simulink library "lib_FDM"  (R2019b)
settings: Solver=VariableStepAuto  StartTime=0.0  StopTime=10.0  RelTol=1e-3
values from neighbouring files (symbols this model uses):
  d = config.d_m    [computeTF.m]
undefined symbols (not defined in the file or in its folder): c_b_WGS, c_flat, c_grav, c_rot, c_rsma, Cd0, Cdcl, Cdcl2, Cl0, Cla, Cld, Cma, Cmd, Cmq, Cnb, Cnd, Cnr, Cra, Crd, Crp, Cy0, Cyb, Cyd, dmdt, Earth, HIL_Data, InitThrust, launchPos, me, mf, mp, Sref, tb, TF, theta0, WGS84
libraries: simulink_extras x14, $bdroot x7, simulink x5, lib_Fin_Deflections x3, aerolibasang x2, sharedtransform x1, aerolibtransform2 x1, aerolibbdyn x1, aerolibatmos2 x1, aerolibutil x1, aerolib6dof2 x1
(part 3 of 8)

== system lib_FDM/FDM/FDM_Basic/State_Integration/VEL_Integrator ==
  Simulation_Control : Inport  OutDataTypeStr=Bus: Simulation_Ctrl_Bus
  Initial_States : Inport  Port=2  OutDataTypeStr=Bus: States_Bus
  ax_mDs2 : Inport  Port=3
  ay_mDs2 : Inport  Port=4
  az_mDs2 : Inport  Port=5
  Bus Selector : BusSelector  OutputSignals=run,reset
  Bus Selector1 : BusSelector  OutputSignals=Rigid_Body_States.Translation_States.VEL_u_K_R_E_B_mDs
  Bus Selector2 : BusSelector  OutputSignals=Rigid_Body_States.Translation_States.VEL_v_K_R_E_B_mDs
  Bus Selector3 : BusSelector  OutputSignals=Rigid_Body_States.Translation_States.VEL_w_K_R_E_B_mDs
  Data Type Conversion : DataTypeConversion  OutDataTypeStr=double
  Integrator : Integrator  ExternalReset=rising  InitialConditionSource=external
  Integrator1 : Integrator  ExternalReset=rising  InitialConditionSource=external
  Integrator2 : Integrator  ExternalReset=rising  InitialConditionSource=external
  Product : Product
  Product1 : Product
  Product2 : Product
  u_mDs : Outport  VectorParamsAs1DForOutWhenUnconnected=off
  v_mDs : Outport  Port=2  VectorParamsAs1DForOutWhenUnconnected=off
  w_mDs : Outport  Port=3  VectorParamsAs1DForOutWhenUnconnected=off
  wires:
  Simulation_Control/1 -> Bus Selector/1
  Bus Selector/1 -> Data Type Conversion/1  "<run>"
  Data Type Conversion/1 -> Product/2, Product1/2, Product2/2
  Product/1 -> Integrator/1
  az_mDs2/1 -> Product2/1
  ay_mDs2/1 -> Product1/1
  ax_mDs2/1 -> Product/1
  Bus Selector/2 -> Integrator2/2, Integrator1/2, Integrator/2  "<reset>"
  Bus Selector1/1 -> Integrator/3  "<VEL_u_K_R_E_B_mDs>"
  Product1/1 -> Integrator1/1
  Initial_States/1 -> Bus Selector3/1, Bus Selector2/1, Bus Selector1/1
  Product2/1 -> Integrator2/1
  Integrator/1 -> u_mDs/1  "u"
  Integrator1/1 -> v_mDs/1  "v"
  Integrator2/1 -> w_mDs/1  "w"
  Bus Selector3/1 -> Integrator2/3  "<VEL_w_K_R_E_B_mDs>"
  Bus Selector2/1 -> Integrator1/3  "<VEL_v_K_R_E_B_mDs>"

== system lib_FDM/FDM/FDM_Linear/Motion_Kinematics/Drag ==
  alpha : Inport
  beta : Inport  Port=2
  Enable : EnablePort
  Constant : Constant  Value=-1
  Constant1 : Constant  Value=-1
  Constant2 : Constant  Value=-1
  Terminator : Terminator
  Terminator1 : Terminator
  acc_x_drag_mDs2 : Outport  OutputWhenDisabled=reset  InitialOutput=0  VectorParamsAs1DForOutWhenUnconnected=off
  acc_y_drag_mDs2 : Outport  Port=2  OutputWhenDisabled=reset  InitialOutput=0  VectorParamsAs1DForOutWhenUnconnected=off
  acc_z_drag_mDs2 : Outport  Port=3  OutputWhenDisabled=reset  InitialOutput=0  VectorParamsAs1DForOutWhenUnconnected=off
  wires:
  alpha/1 -> Terminator/1
  beta/1 -> Terminator1/1
  Constant/1 -> acc_x_drag_mDs2/1
  Constant1/1 -> acc_y_drag_mDs2/1
  Constant2/1 -> acc_z_drag_mDs2/1

== system lib_FDM/FDM/FDM_Linear/Motion_Kinematics/Gravity ==
  note: derived from transformation matrix NED to Body
  note: for decoupling, set phi to zero??!!!
  phi : Inport
  theta : Inport  Port=2
  psi : Inport  Port=3
  Enable : EnablePort
  Constant1 : Constant  Value=FDM.Environment_Data.gravity_mDs2
  MATLAB Function : MATLAB Function  TreatAsAtomicUnit=on
  acc_x_grav_mDs : Outport  OutputWhenDisabled=reset  InitialOutput=0  VectorParamsAs1DForOutWhenUnconnected=off
  acc_y_grav_mDs : Outport  Port=2  OutputWhenDisabled=reset  InitialOutput=0  VectorParamsAs1DForOutWhenUnconnected=off
  acc_z_grav_mDs : Outport  Port=3  OutputWhenDisabled=reset  InitialOutput=0  VectorParamsAs1DForOutWhenUnconnected=off
  wires:
  Constant1/1 -> MATLAB Function/1(g)
  phi/1 -> MATLAB Function/2(phi)
  theta/1 -> MATLAB Function/3(theta)
  psi/1 -> MATLAB Function/4(psi)
  MATLAB Function/1(acc_x) -> acc_x_grav_mDs/1
  MATLAB Function/2(acc_y) -> acc_y_grav_mDs/1
  MATLAB Function/3(acc_z) -> acc_z_grav_mDs/1

== system lib_FDM/FDM/FDM_Linear/Motion_Kinematics/NED2PosWGS84Dot ==
  note: derived from Scriptum
  mue_rad : Inport
  h_m : Inport  Port=2
  x_dot_NED_mDs : Inport  Port=3
  y_dot_NED_mDs : Inport  Port=4
  z_dot_NED_mDs : Inport  Port=5
  MATLAB Function : MATLAB Function  TreatAsAtomicUnit=on
  lambda_dot_radDs : Outport  VectorParamsAs1DForOutWhenUnconnected=off
  mue_dot_radDs : Outport  Port=2  VectorParamsAs1DForOutWhenUnconnected=off
  h_dot_mDs : Outport  Port=3  VectorParamsAs1DForOutWhenUnconnected=off
  wires:
  h_m/1 -> MATLAB Function/5(h)
  mue_rad/1 -> MATLAB Function/4(mue)
  z_dot_NED_mDs/1 -> MATLAB Function/3(z_dot_NED)
  y_dot_NED_mDs/1 -> MATLAB Function/2(y_dot_NED)
  x_dot_NED_mDs/1 -> MATLAB Function/1(x_dot_NED)
  MATLAB Function/3(h_dot) -> h_dot_mDs/1
  MATLAB Function/2(mue_dot) -> mue_dot_radDs/1
  MATLAB Function/1(lambda_dot) -> lambda_dot_radDs/1

== system lib_FDM/FDM/FDM_Linear/Motion_Kinematics/Propulsion ==
  Motor_Ignition_flg : Inport
  Enable : EnablePort
  Add : Sum  Inputs=-+
  Clock : Clock
  Compare To Constant : simulink/Logic and Bit Operations/Compare To Constant  relop=<  const=FDM.Configuration_Data.Propulsion.burntime_s  OutDataTypeStr=boolean
  Logical Operator : Logic  Operator=NOT  AllPortsSameDT=off  OutDataTypeStr=boolean
  Logical Operator1 : Logic  Operator=OR  AllPortsSameDT=off  OutDataTypeStr=boolean
  Logical Operator2 : Logic  AllPortsSameDT=off  OutDataTypeStr=boolean
  Subsystem : Subsystem
  hold_time : Subsystem
  lock : Memory
  F_x_prop_N : Outport  VectorParamsAs1DForOutWhenUnconnected=off
  motor_state_perc_dot : Outport  Port=2  OutputWhenDisabled=reset  InitialOutput=0  VectorParamsAs1DForOutWhenUnconnected=off
  wires:
  Motor_Ignition_flg/1 -> Logical Operator1/1
  Logical Operator1/1 -> lock/1, Logical Operator/1, Logical Operator2/1
  lock/1 -> Logical Operator1/2
  Logical Operator/1 -> hold_time/Enable
  hold_time/1(exec_time_hold_s) -> Add/1
  Clock/1 -> Add/2
  Add/1 -> Compare To Constant/1, Subsystem/1(runtime)
  Subsystem/1(thrust) -> F_x_prop_N/1
  Subsystem/2(state_percentage_change) -> motor_state_perc_dot/1
  Compare To Constant/1 -> Logical Operator2/2
  Logical Operator2/1 -> Subsystem/Enable

== system lib_FDM/FDM/FDM_Linear/Motion_Kinematics/pqr2EulerDot ==
  ATT : Inport  OutDataTypeStr=Bus: ATT_Euler_Bus
  p : Inport  Port=2
  q : Inport  Port=3
  r : Inport  Port=4
  Add : Sum  Inputs=+++
  Add1 : Sum
  Add2 : Sum
  Bus Selector : BusSelector  OutputSignals=ATT_Phi_rad,ATT_Theta_rad
  Divide : Product  Inputs=*/
  Divide1 : Product  Inputs=*/
  Fcn1 : Fcn  Expr=-sin(u)
  Fcn{6,8,10..12} (5 alike) : Fcn  Expr=cos(u)
  Fcn4 : Fcn  Expr=sin(u)
  Fcn5 : Fcn  Expr=tan(u)
  Fcn7 : Fcn  Expr=tan(u)
  Fcn9 : Fcn  Expr=sin(u)
  Multiply{,1..7} (8 alike) : Product
  phi_dot : Outport  VectorParamsAs1DForOutWhenUnconnected=off
  theta_dot : Outport  Port=2  VectorParamsAs1DForOutWhenUnconnected=off
  psi_dot : Outport  Port=3  VectorParamsAs1DForOutWhenUnconnected=off
  wires:
  ATT/1 -> Bus Selector/1
  Add2/1 -> psi_dot/1
  Add1/1 -> theta_dot/1
  Add/1 -> phi_dot/1
  Fcn4/1 -> Multiply/1
  Fcn5/1 -> Multiply/2
  p/1 -> Add/1
  Bus Selector/1 -> Fcn1/1, Fcn8/1, Fcn6/1, Fcn4/1, Fcn11/1, Fcn9/1  "<ATT_Phi_rad>"
  Bus Selector/2 -> Fcn7/1, Fcn5/1, Fcn12/1, Fcn10/1  "<ATT_Theta_rad>"
  Fcn6/1 -> Multiply1/1
  Fcn7/1 -> Multiply1/2
  Fcn9/1 -> Divide/1
  Fcn10/1 -> Divide/2
  Fcn11/1 -> Divide1/1
  Fcn12/1 -> Divide1/2
  Multiply/1 -> Multiply2/2
  q/1 -> Multiply2/1, Multiply6/1, Multiply4/2
  Multiply2/1 -> Add/2
  Multiply1/1 -> Multiply3/2
  r/1 -> Multiply3/1, Multiply7/1, Multiply5/2
  Multiply3/1 -> Add/3
  Fcn8/1 -> Multiply4/1
  Fcn1/1 -> Multiply5/1
  Multiply4/1 -> Add1/1
  Multiply5/1 -> Add1/2
  Divide/1 -> Multiply6/2
  Divide1/1 -> Multiply7/2
  Multiply6/1 -> Add2/1
  Multiply7/1 -> Add2/2

== system lib_FDM/FDM/FDM_Linear/Motion_Kinematics/uvw2PosNEDDot ==
  note: for decoupling, set phi to zero??!!!
  note: derived from Rotation Matrix Body Frame to NED Frame
  u : Inport
  v : Inport  Port=2
  w : Inport  Port=3
  ATT : Inport  Port=4  OutDataTypeStr=Bus: ATT_Euler_Bus
  Bus Selector : BusSelector  OutputSignals=ATT_Phi_rad,ATT_Theta_rad,ATT_Psi_rad
  MATLAB Function : MATLAB Function  TreatAsAtomicUnit=on
  MATLAB Function1 : MATLAB Function  TreatAsAtomicUnit=on
  MATLAB Function2 : MATLAB Function  TreatAsAtomicUnit=on
  x_dot_mDs : Outport  VectorParamsAs1DForOutWhenUnconnected=off
  y_dot_mDs : Outport  Port=2  VectorParamsAs1DForOutWhenUnconnected=off
  z_dot_mDs : Outport  Port=3  VectorParamsAs1DForOutWhenUnconnected=off
  wires:
  ATT/1 -> Bus Selector/1
  u/1 -> MATLAB Function2/1(u), MATLAB Function1/1(u), MATLAB Function/1(u)
  v/1 -> MATLAB Function2/2(v), MATLAB Function1/2(v), MATLAB Function/2(v)
  w/1 -> MATLAB Function2/3(w), MATLAB Function1/3(w), MATLAB Function/3(w)
  Bus Selector/1 -> MATLAB Function2/4(phi), MATLAB Function1/4(phi), MATLAB Function/4(phi)  "<ATT_Phi_rad>"
  Bus Selector/2 -> MATLAB Function2/5(theta), MATLAB Function1/5(theta), MATLAB Function/5(theta)  "<ATT_Theta_rad>"
  Bus Selector/3 -> MATLAB Function1/6(psi), MATLAB Function/6(psi)  "<ATT_Psi_rad>"
  MATLAB Function/1(N_dot) -> x_dot_mDs/1
  MATLAB Function1/1(E_dot) -> y_dot_mDs/1
  MATLAB Function2/1(D_dot) -> z_dot_mDs/1

== system lib_FDM/FDM/FDM_Linear/State_Integration/ATT_Integration ==
  Simulation_Control : Inport  OutDataTypeStr=Bus: Simulation_Ctrl_Bus
  Initial_States : Inport  Port=2  OutDataTypeStr=Bus: States_Bus
  phi_dot_radDs : Inport  Port=3
  theta_dot_radDs : Inport  Port=4
  psi_dot_radDs : Inport  Port=5
  Bus Selector : BusSelector  OutputSignals=run,reset
  Bus Selector1 : BusSelector  OutputSignals=Rigid_Body_States.Attitude_States.ATT_Euler.ATT_Phi_rad
  Bus Selector2 : BusSelector  OutputSignals=Rigid_Body_States.Attitude_States.ATT_Euler.ATT_Theta_rad
  Bus Selector3 : BusSelector  OutputSignals=Rigid_Body_States.Attitude_States.ATT_Euler.ATT_Psi_rad
  Data Type Conversion : DataTypeConversion  OutDataTypeStr=double
  Integrator : Integrator  ExternalReset=rising  InitialConditionSource=external
  Integrator1 : Integrator  ExternalReset=rising  InitialConditionSource=external
  Integrator2 : Integrator  ExternalReset=rising  InitialConditionSource=external
  Product : Product
  Product1 : Product
  Product2 : Product
  phi_rad : Outport  VectorParamsAs1DForOutWhenUnconnected=off
  theta_rad : Outport  Port=2  VectorParamsAs1DForOutWhenUnconnected=off
  psi_rad : Outport  Port=3  VectorParamsAs1DForOutWhenUnconnected=off
  wires:
  Simulation_Control/1 -> Bus Selector/1
  Bus Selector/1 -> Data Type Conversion/1  "<run>"
  Data Type Conversion/1 -> Product/2, Product1/2, Product2/2
  Product/1 -> Integrator/1
  psi_dot_radDs/1 -> Product2/1
  theta_dot_radDs/1 -> Product1/1
  phi_dot_radDs/1 -> Product/1
  Bus Selector/2 -> Integrator2/2, Integrator1/2, Integrator/2  "<reset>"
  Bus Selector1/1 -> Integrator/3  "<ATT_Phi_rad>"
  Product1/1 -> Integrator1/1
  Initial_States/1 -> Bus Selector3/1, Bus Selector2/1, Bus Selector1/1
  Product2/1 -> Integrator2/1
  Integrator/1 -> phi_rad/1
  Integrator1/1 -> theta_rad/1
  Integrator2/1 -> psi_rad/1
  Bus Selector3/1 -> Integrator2/3  "<ATT_Psi_rad>"
  Bus Selector2/1 -> Integrator1/3  "<ATT_Theta_rad>"

== system lib_FDM/FDM/FDM_Linear/State_Integration/Mass_Balance ==
  note: linear interpolation between initial and burnout values of inertia and mass
  motor_state_perc : Inport
  Add{,1..3} (4 alike) : Sum
  Constant : Constant  Value=FDM.Configuration_Data.mass_preburn_kg-FDM.Configuration_Data.mass_kg
  Constant1 : Constant  Value=FDM.Configuration_Data.mass_kg
  Constant2 : Constant  Value=FDM.Configuration_Data.I_x_kgDm2
  Constant3 : Constant  Value=FDM.Configuration_Data.I_x_preburn_kgDm2-FDM.Configuration_Data.I_x_kgDm2
  Constant4 : Constant  Value=FDM.Configuration_Data.I_y_kgDm2
  Constant5 : Constant  Value=FDM.Configuration_Data.I_y_preburn_kgDm2-FDM.Configuration_Data.I_y_kgDm2
  Constant6 : Constant  Value=FDM.Configuration_Data.I_z_kgDm2
  Constant7 : Constant  Value=FDM.Configuration_Data.I_z_preburn_kgDm2-FDM.Configuration_Data.I_z_kgDm2
  Multiply{,1..3} (4 alike) : Product
  mass_kg : Outport  VectorParamsAs1DForOutWhenUnconnected=off
  I_x_kgm2 : Outport  Port=2  VectorParamsAs1DForOutWhenUnconnected=off
  I_y_kgm2 : Outport  Port=3  VectorParamsAs1DForOutWhenUnconnected=off
  I_z_kgm2 : Outport  Port=4  VectorParamsAs1DForOutWhenUnconnected=off
  wires:
  Constant1/1 -> Add/1
  Constant/1 -> Multiply/2
  Multiply/1 -> Add/2
  motor_state_perc/1 -> Multiply1/1, Multiply2/1, Multiply3/1, Multiply/1
  Add/1 -> mass_kg/1
  Constant3/1 -> Multiply1/2
  Multiply1/1 -> Add1/2
  Constant2/1 -> Add1/1
  Constant5/1 -> Multiply2/2
  Constant4/1 -> Add2/1
  Multiply2/1 -> Add2/2
  Constant6/1 -> Add3/1
  Constant7/1 -> Multiply3/2
  Multiply3/1 -> Add3/2
  Add1/1 -> I_x_kgm2/1
  Add2/1 -> I_y_kgm2/1
  Add3/1 -> I_z_kgm2/1

== system lib_FDM/FDM/FDM_Linear/State_Integration/Motor_State_Integration ==
  Simulation_Control : Inport  OutDataTypeStr=Bus: Simulation_Ctrl_Bus
  Initial_States : Inport  Port=2  OutDataTypeStr=Bus: States_Bus
  motor_state_dot_percDs : Inport  Port=3
  Bus Selector2 : BusSelector  OutputSignals=Airframe_States.motor_state_perc
  Bus Selector3 : BusSelector  OutputSignals=run,reset
  Data Type Conversion : DataTypeConversion  OutDataTypeStr=double
  Integrator : Integrator  ExternalReset=rising  InitialConditionSource=external
  Multiply : Product
  motor_state_perc : Outport  VectorParamsAs1DForOutWhenUnconnected=off
  wires:
  Bus Selector2/1 -> Integrator/3  "<motor_state_perc>"
  Bus Selector3/2 -> Integrator/2  "<reset>"
  Bus Selector3/1 -> Data Type Conversion/1  "<run>"
  motor_state_dot_percDs/1 -> Multiply/1
  Integrator/1 -> motor_state_perc/1
  Multiply/1 -> Integrator/1
  Simulation_Control/1 -> Bus Selector3/1
  Initial_States/1 -> Bus Selector2/1
  Data Type Conversion/1 -> Multiply/2

== system lib_FDM/FDM/FDM_Linear/State_Integration/POS_NED_Integrator ==
  Simulation_Control : Inport  OutDataTypeStr=Bus: Simulation_Ctrl_Bus
  Initial_States : Inport  Port=2  OutDataTypeStr=Bus: States_Bus
  x_dot_mDs : Inport  Port=3
  y_dot_mDs : Inport  Port=4
  z_dot_mDs : Inport  Port=5
  Bus Selector : BusSelector  OutputSignals=run,reset
  Bus Selector1 : BusSelector  OutputSignals=Rigid_Body_States.Position_States.POS_NED.POS_x_NED_m
  Bus Selector2 : BusSelector  OutputSignals=Rigid_Body_States.Position_States.POS_NED.POS_y_NED_m
  Bus Selector3 : BusSelector  OutputSignals=Rigid_Body_States.Position_States.POS_NED.POS_z_NED_m
  Data Type Conversion : DataTypeConversion  OutDataTypeStr=double
  Integrator : Integrator  ExternalReset=rising  InitialConditionSource=external
  Integrator1 : Integrator  ExternalReset=rising  InitialConditionSource=external
  Integrator2 : Integrator  ExternalReset=rising  InitialConditionSource=external
  Product : Product
  Product1 : Product
  Product2 : Product
  x_m : Outport  VectorParamsAs1DForOutWhenUnconnected=off
  y_m : Outport  Port=2  VectorParamsAs1DForOutWhenUnconnected=off
  z_m : Outport  Port=3  VectorParamsAs1DForOutWhenUnconnected=off
  wires:
  Simulation_Control/1 -> Bus Selector/1
  Bus Selector/1 -> Data Type Conversion/1  "<run>"
  Data Type Conversion/1 -> Product/2, Product1/2, Product2/2
  Product/1 -> Integrator/1
  z_dot_mDs/1 -> Product2/1
  y_dot_mDs/1 -> Product1/1
  x_dot_mDs/1 -> Product/1
  Bus Selector/2 -> Integrator2/2, Integrator1/2, Integrator/2  "<reset>"
  Bus Selector1/1 -> Integrator/3  "<POS_x_NED_m>"
  Product1/1 -> Integrator1/1
  Initial_States/1 -> Bus Selector3/1, Bus Selector2/1, Bus Selector1/1
  Product2/1 -> Integrator2/1
  Integrator/1 -> x_m/1
  Integrator1/1 -> y_m/1
  Integrator2/1 -> z_m/1
  Bus Selector3/1 -> Integrator2/3  "<POS_z_NED_m>"
  Bus Selector2/1 -> Integrator1/3  "<POS_y_NED_m>"

== system lib_FDM/FDM/FDM_Linear/State_Integration/POS_WGS84_Integrator ==
  Simulation_Control : Inport  OutDataTypeStr=Bus: Simulation_Ctrl_Bus
  Initial_States : Inport  Port=2  OutDataTypeStr=Bus: States_Bus
  lambda_dot_radDs : Inport  Port=3
  mue_dot_radDs : Inport  Port=4
  h_dot_mDs : Inport  Port=5
  Bus Selector : BusSelector  OutputSignals=run,reset
  Bus Selector1 : BusSelector  OutputSignals=Rigid_Body_States.Position_States.POS_WGS84.POS_lambda_WGS84_rad
  Bus Selector2 : BusSelector  OutputSignals=Rigid_Body_States.Position_States.POS_WGS84.POS_mue_WGS84_rad
  Bus Selector3 : BusSelector  OutputSignals=Rigid_Body_States.Position_States.POS_WGS84.POS_h_WGS84_m
  Data Type Conversion : DataTypeConversion  OutDataTypeStr=double
  Integrator : Integrator  ExternalReset=rising  InitialConditionSource=external
  Integrator1 : Integrator  ExternalReset=rising  InitialConditionSource=external
  Integrator2 : Integrator  ExternalReset=rising  InitialConditionSource=external
  Product : Product
  Product1 : Product
  Product2 : Product
  lambda_rad : Outport  VectorParamsAs1DForOutWhenUnconnected=off
  mue_rad : Outport  Port=2  VectorParamsAs1DForOutWhenUnconnected=off
  h_m : Outport  Port=3  VectorParamsAs1DForOutWhenUnconnected=off
  wires:
  Simulation_Control/1 -> Bus Selector/1
  Bus Selector/1 -> Data Type Conversion/1  "<run>"
  Data Type Conversion/1 -> Product/2, Product1/2, Product2/2
  Product/1 -> Integrator/1
  h_dot_mDs/1 -> Product2/1
  mue_dot_radDs/1 -> Product1/1
  lambda_dot_radDs/1 -> Product/1
  Bus Selector/2 -> Integrator2/2, Integrator1/2, Integrator/2  "<reset>"
  Bus Selector1/1 -> Integrator/3  "<POS_lambda_WGS84_rad>"
  Product1/1 -> Integrator1/1
  Initial_States/1 -> Bus Selector3/1, Bus Selector2/1, Bus Selector1/1
  Product2/1 -> Integrator2/1
  Integrator/1 -> lambda_rad/1
  Integrator1/1 -> mue_rad/1
  Integrator2/1 -> h_m/1
  Bus Selector3/1 -> Integrator2/3  "<POS_h_WGS84_m>"
  Bus Selector2/1 -> Integrator1/3  "<POS_mue_WGS84_rad>"

== system lib_FDM/FDM/FDM_Linear/State_Integration/VEL_Integrator ==
  Simulation_Control : Inport  OutDataTypeStr=Bus: Simulation_Ctrl_Bus
  Initial_States : Inport  Port=2  OutDataTypeStr=Bus: States_Bus
  ax_mDs2 : Inport  Port=3
  ay_mDs2 : Inport  Port=4
  az_mDs2 : Inport  Port=5
  Bus Selector : BusSelector  OutputSignals=run,reset
  Bus Selector1 : BusSelector  OutputSignals=Rigid_Body_States.Translation_States.VEL_u_K_R_E_B_mDs
  Bus Selector2 : BusSelector  OutputSignals=Rigid_Body_States.Translation_States.VEL_v_K_R_E_B_mDs
  Bus Selector3 : BusSelector  OutputSignals=Rigid_Body_States.Translation_States.VEL_w_K_R_E_B_mDs
  Data Type Conversion : DataTypeConversion  OutDataTypeStr=double
  Integrator : Integrator  ExternalReset=rising  InitialConditionSource=external
  Integrator1 : Integrator  ExternalReset=rising  InitialConditionSource=external
  Integrator2 : Integrator  ExternalReset=rising  InitialConditionSource=external
  Product : Product
  Product1 : Product
  Product2 : Product
  u_mDs : Outport  VectorParamsAs1DForOutWhenUnconnected=off
  v_mDs : Outport  Port=2  VectorParamsAs1DForOutWhenUnconnected=off
  w_mDs : Outport  Port=3  VectorParamsAs1DForOutWhenUnconnected=off
  wires:
  Simulation_Control/1 -> Bus Selector/1
  Bus Selector/1 -> Data Type Conversion/1  "<run>"
  Data Type Conversion/1 -> Product/2, Product1/2, Product2/2
  Product/1 -> Integrator/1
  az_mDs2/1 -> Product2/1
  ay_mDs2/1 -> Product1/1
  ax_mDs2/1 -> Product/1
  Bus Selector/2 -> Integrator2/2, Integrator1/2, Integrator/2  "<reset>"
  Bus Selector1/1 -> Integrator/3  "<VEL_u_K_R_E_B_mDs>"
  Product1/1 -> Integrator1/1
  Initial_States/1 -> Bus Selector3/1, Bus Selector2/1, Bus Selector1/1
  Product2/1 -> Integrator2/1
  Integrator/1 -> u_mDs/1  "u"
  Integrator1/1 -> v_mDs/1  "v"
  Integrator2/1 -> w_mDs/1  "w"
  Bus Selector3/1 -> Integrator2/3  "<VEL_w_K_R_E_B_mDs>"
  Bus Selector2/1 -> Integrator1/3  "<VEL_v_K_R_E_B_mDs>"

== system lib_FDM/FDM/FDM_Sophisticated/Subsystem/control_allocation ==
  fin_cmd : Inport
  Constant7 : Constant  Value=HIL_Data.FDM.soph.bus1.Tr4r3
  Product : Product  Multiplication=Matrix(*)
  siB_cmd : Outport  VectorParamsAs1DForOutWhenUnconnected=off
  wires:
  Constant7/1 -> Product/1
  fin_cmd/1 -> Product/2
  Product/1 -> siB_cmd/1  "siB_cmd"

== system lib_FDM/FDM/FDM_Sophisticated/aerodynamics/aerodynamic_via_lookup ==
  pBSB : Inport
  qdynB : Inport  Port=2
  MaB : Inport  Port=3
  alB : Inport  Port=4
  beB : Inport  Port=5
  hBE : Inport  Port=6
  wBIB_star : Inport  Port=7
  afinB : Inport  Port=8
  flag_I_prp : Inport  Port=9
  Bus Creator : BusCreator  Inputs=2
  calc_aero_coefficients : Subsystem
  calc_aero_for_mom : Subsystem
  calc_derivatives : Subsystem
  transform_rad2deg_al_be : Subsystem
  transform_rad2deg_fin : Subsystem
  transform_rad2deg_rates : Subsystem
  aero_bus : Outport  VectorParamsAs1DForOutWhenUnconnected=off
  wires:
  transform_rad2deg_al_be/2(beB_deg) -> calc_derivatives/4(beB)
  transform_rad2deg_al_be/1(alB_deg) -> calc_derivatives/3(alB)
  beB/1 -> transform_rad2deg_al_be/2(beB)
  afinB/1 -> transform_rad2deg_fin/1(afinB)
  qdynB/1 -> calc_aero_for_mom/3(qdynB)
  calc_aero_for_mom/2(MBAB) -> Bus Creator/2
  calc_aero_coefficients/6(Cn) -> calc_aero_for_mom/9(Cn)
  calc_aero_coefficients/1(Cx) -> calc_aero_for_mom/4(Cx)
  calc_aero_coefficients/5(Cm) -> calc_aero_for_mom/8(Cm)
  calc_derivatives/4(Cl_deriv) -> calc_aero_coefficients/4(Cl_deriv)
  calc_aero_coefficients/3(Cz) -> calc_aero_for_mom/6(Cz)
  hBE/1 -> calc_aero_for_mom/1(hBE), calc_derivatives/1(hBE)
  flag_I_prp/1 -> calc_aero_coefficients/13(flag_base_drag)
  calc_derivatives/6(Cn_deriv) -> calc_aero_coefficients/6(Cn_deriv)
  wBIB_star/1 -> transform_rad2deg_rates/1(wBIB_star)
  calc_derivatives/3(Cz_deriv) -> calc_aero_coefficients/3(Cz_deriv)
  pBSB/1 -> calc_aero_for_mom/2(pBSB)
  transform_rad2deg_rates/2(qBIB_star_deg) -> calc_aero_coefficients/11(qBIB_star)
  transform_rad2deg_rates/3(rBIB_star_deg) -> calc_aero_coefficients/12(rBIB_star)
  Bus Creator/1 -> aero_bus/1  "aero_bus"
  calc_aero_coefficients/2(Cy) -> calc_aero_for_mom/5(Cy)
  calc_derivatives/5(Cm_deriv) -> calc_aero_coefficients/5(Cm_deriv)
  calc_derivatives/2(Cy_deriv) -> calc_aero_coefficients/2(Cy_deriv)
  transform_rad2deg_rates/1(pBIB_star_deg) -> calc_aero_coefficients/10(pBIB_star)
  transform_rad2deg_fin/3(xiB_deg) -> calc_aero_coefficients/9(xiB_deg)
  transform_rad2deg_fin/2(zeB_deg) -> calc_aero_coefficients/8(zeB_deg), calc_derivatives/6(zeB_deg)
  alB/1 -> transform_rad2deg_al_be/1(alB)
  transform_rad2deg_fin/1(etB_deg) -> calc_derivatives/5(etB_deg), calc_aero_coefficients/7(etB_deg)
  calc_derivatives/1(Cx_deriv) -> calc_aero_coefficients/1(Cx_deriv)
  calc_aero_for_mom/1(FBAB) -> Bus Creator/1
  MaB/1 -> calc_derivatives/2(MaB)
  calc_aero_coefficients/4(Cl) -> calc_aero_for_mom/7(Cl)

== system lib_FDM/FDM/FDM_Sophisticated/aerodynamics/logic_base_drag ==
  env_glbl : Inport
  Bus Selector1 : BusSelector  OutputSignals=T_sim_glbl,T_sim_lnch
  Constant : Constant  Value=HIL_Data.FDM.soph.bus1.t_prp2(end)
  MATLAB Function : MATLAB Function  TreatAsAtomicUnit=on
  Subtract : Sum  Inputs=+-
  flag_base_drag : Outport  VectorParamsAs1DForOutWhenUnconnected=off
  wires:
  env_glbl/1 -> Bus Selector1/1
  Bus Selector1/2 -> Subtract/2  "<T_sim_lnch>"
  Bus Selector1/1 -> Subtract/1  "<T_sim_glbl>"
  MATLAB Function/1(flag_base_drag) -> flag_base_drag/1  "flag_base_drag"
  Constant/1 -> MATLAB Function/2(t_prp2)
  Subtract/1 -> MATLAB Function/1(u)

== system lib_FDM/FDM/FDM_Sophisticated/environment/WGS84_Gravitation ==
  lon : Inport  PortDimensions=1
  lat : Inport  Port=2  PortDimensions=1
  h : Inport  Port=3  PortDimensions=1
  Assertion : Assertion  AssertionFailFcn="error('WGS84 Gravitationsmodell: Die Werte des Eingangs \"h\" muessen groesser als 0 sein')"
  Assertion1 : Assertion  AssertionFailFcn="error('WGS84 Gravitationsmodell: Die Werte des Eingangs \"Long\" muessen zwischen -180 und +180 liegen')"
  Assertion2 : Assertion  AssertionFailFcn="error('WGS84 Gravitationsmodell: Die Werte des Eingangs \"Lat\" muessen zwischen -90 und +90 liegen')"
  Compare To Constant : simulink/Logic and Bit Operations/Compare To Constant  relop=>=  const=0  OutDataTypeStr=boolean
      settings: SourceProductName=ISim Simulink Block Set
  Interval Test : simulink/Logic and Bit Operations/Interval Test  IntervalClosedRight=on  uplimit=pi  IntervalClosedLeft=on  lowlimit=-pi  OutDataTypeStr=boolean
      settings: SourceProductName=ISim Simulink Block Set
  Interval Test1 : simulink/Logic and Bit Operations/Interval Test  IntervalClosedRight=on  uplimit=pi/2  IntervalClosedLeft=on  lowlimit=-pi/2  OutDataTypeStr=boolean
      settings: SourceProductName=ISim Simulink Block Set
  WGS84_2_ECEF : Subsystem
  WGS84_Gravity_Implementation : MATLAB Function  TreatAsAtomicUnit=on
  gE : Outport  PortDimensions=3  VectorParamsAs1DForOutWhenUnconnected=off
  wires:
  WGS84_Gravity_Implementation/1(gamma_R) -> gE/1  "gE"
  h/1 -> Compare To Constant/1, WGS84_2_ECEF/1(h)  "h"
  lon/1 -> WGS84_2_ECEF/2(lon), Interval Test/1, WGS84_Gravity_Implementation/3(long_rad)  "lon"
  lat/1 -> WGS84_2_ECEF/3(lat), Interval Test1/1, WGS84_Gravity_Implementation/2(lat_rad)  "lat"
  WGS84_2_ECEF/1(pE) -> WGS84_Gravity_Implementation/1(pE)  "pE"
  Compare To Constant/1 -> Assertion/1
  Interval Test/1 -> Assertion1/1
  Interval Test1/1 -> Assertion2/1

== system lib_FDM/FDM/FDM_Sophisticated/environment/atmosphere_static_ISO_2533 ==
  hBE : Inport
  env_glbl : Inport  Port=2
  Bus Creator1 : BusCreator  Inputs=6
  Bus Selector1 : BusSelector  OutputSignals=e_Tmp,e_pa
  Saturation : Saturate  UpperLimit=HIL_Data.FDM.soph.bus2.c_h_geope  LowerLimit=HIL_Data.FDM.soph.bus2.c_h_geop0
      settings: AttributesFormatString=|
      | %<UpperLimit>
      | %<LowerLimit>
  density : Subsystem
  geopot_height : Subsystem  mask{mean_earth_radius=HIL_Data.FDM.soph.bus2.c_r0}
      mask prompts: mean_earth_radius "Mean Earth Radius WGS 84 [m]"
      mask TypeOptions mean_earth_radius: mean_earth_radius/Value
  speed_of_sound : Subsystem
  tmp_and_pressure_ISO_2533 : Subsystem
  atm_stat : Outport  VectorParamsAs1DForOutWhenUnconnected=off
  wires:
  Saturation/1 -> tmp_and_pressure_ISO_2533/1(h_geop), Bus Creator1/2  "h_geop"
  hBE/1 -> geopot_height/1(hBE), Bus Creator1/1
  density/1(rho) -> Bus Creator1/5
  tmp_and_pressure_ISO_2533/2(pa) -> density/2(pa), Bus Creator1/6
  tmp_and_pressure_ISO_2533/1(Tmp) -> density/1(Tmp), Bus Creator1/4, speed_of_sound/1(Tmp)
  Bus Creator1/1 -> atm_stat/1  "atm_stat_bus"
  Bus Selector1/1 -> tmp_and_pressure_ISO_2533/2(e_Tmp)  "<e_Tmp>"
  geopot_height/1(h_geop) -> Saturation/1
  Bus Selector1/2 -> tmp_and_pressure_ISO_2533/3(e_pa)  "<e_pa>"
  env_glbl/1 -> Bus Selector1/1
  speed_of_sound/1(sos) -> Bus Creator1/3

== system lib_FDM/FDM/FDM_Sophisticated/environment/convert_to_local_frame ==
  gE : Inport
  Constant1 : Constant  Value=0
  Dot Product : DotProduct  InputSameDT=on  OutDataTypeStr=Inherit: Inherit via internal rule
  Sqrt : Sqrt  SaturateOnIntegerOverflow=on
  Vector Concatenate : Concatenate  NumInputs=3  Mode=Multidimensional array
  gBG : Outport  VectorParamsAs1DForOutWhenUnconnected=off
  wires:
  Dot Product/1 -> Sqrt/1
  Vector Concatenate/1 -> gBG/1  "gBG"
  Sqrt/1 -> Vector Concatenate/3
  Constant1/1 -> Vector Concatenate/1, Vector Concatenate/2
  gE/1 -> Dot Product/2, Dot Product/1

== system lib_FDM/FDM/FDM_Sophisticated/fin_actuators/Rudder ==
  siB_c : Inport
  tRRR : Inport  Port=2
  Add : Sum  Inputs=+-
  Add1 : Sum  Inputs=+-
  Add2 : Sum  Inputs=+++
  Constant : Constant  Value=unc_off
  Gain : Gain  Gain=omega^2
  Gain1 : Gain  Gain=unc_scale
  Gain2 : Gain  Gain=2*dmp*omega  Multiplication=Matrix(K*u)
  Gain3 : Gain  Gain=unc_bl
  Integrator : Integrator  ExternalReset=either  InitialCondition=d_siB_0
  Integrator1 : Integrator  InitialCondition=siB_0  LimitOutput=on  UpperSaturationLimit=siB_max  LowerSaturationLimit=siB_min  ShowSaturationPort=on
  Limiting_Acceleration : MATLAB Function  TreatAsAtomicUnit=on
  Limiting_Rate : MATLAB Function  TreatAsAtomicUnit=on
  Saturation : Saturate  UpperLimit=siB_max  LowerLimit=siB_min
  Saturation1 : Saturate  UpperLimit=siB_max  LowerLimit=siB_min
  Sign : Signum
  siB : Outport  VectorParamsAs1DForOutWhenUnconnected=off
  d_siB : Outport  Port=2  VectorParamsAs1DForOutWhenUnconnected=off
  dd_siB : Outport  Port=3  VectorParamsAs1DForOutWhenUnconnected=off
  wires:
  [siB] -> Limiting_Rate/1(siB)
  [siB] -> Limiting_Acceleration/1(siB)
  [d_siB] -> Limiting_Acceleration/2(d_siB)
  siB_c/1 -> Saturation/1  "siB_c"
  Constant/1 -> Add2/1
  Add2/1 -> Saturation1/1
  Saturation/1 -> Add/1
  Integrator/1 -> Gain2/1, Limiting_Rate/2(d_siB)  "d_siB"
  Limiting_Rate/1(d_siB_l) -> Integrator1/1, [d_siB], d_siB/1  "d_siB_l"
  Limiting_Acceleration/1(dd_siB_l) -> dd_siB/1, Integrator/1  "dd_siB_l"
  Add/1 -> Gain/1
  Gain/1 -> Add1/1
  Gain2/1 -> Add1/2
  Add1/1 -> Limiting_Acceleration/3(dd_siB)  "dd_siB"
  Integrator1/1 -> Add/2, Gain1/1  "siB"
  tRRR/1 -> Sign/1  "tRRR"
  Sign/1 -> Gain3/1
  Gain3/1 -> Add2/3
  Gain1/1 -> Add2/2
  Integrator1/2 -> Integrator/2  "sat"
  Saturation1/1 -> [siB], siB/1  "siB"

== system lib_FDM/FDM/FDM_Sophisticated/fin_actuators/Rudder1 ==
  siB_c : Inport
  tRRR : Inport  Port=2
  Add : Sum  Inputs=+-
  Add1 : Sum  Inputs=+-
  Add2 : Sum  Inputs=+++
  Constant : Constant  Value=unc_off
  Gain : Gain  Gain=omega^2
  Gain1 : Gain  Gain=unc_scale
  Gain2 : Gain  Gain=2*dmp*omega  Multiplication=Matrix(K*u)
  Gain3 : Gain  Gain=unc_bl
  Integrator : Integrator  ExternalReset=either  InitialCondition=d_siB_0
  Integrator1 : Integrator  InitialCondition=siB_0  LimitOutput=on  UpperSaturationLimit=siB_max  LowerSaturationLimit=siB_min  ShowSaturationPort=on
  Limiting_Acceleration : MATLAB Function  TreatAsAtomicUnit=on
  Limiting_Rate : MATLAB Function  TreatAsAtomicUnit=on
  Saturation : Saturate  UpperLimit=siB_max  LowerLimit=siB_min
  Saturation1 : Saturate  UpperLimit=siB_max  LowerLimit=siB_min
  Sign : Signum
  siB : Outport  VectorParamsAs1DForOutWhenUnconnected=off
  d_siB : Outport  Port=2  VectorParamsAs1DForOutWhenUnconnected=off
  dd_siB : Outport  Port=3  VectorParamsAs1DForOutWhenUnconnected=off
  wires:
  [siB] -> Limiting_Rate/1(siB)
  [siB] -> Limiting_Acceleration/1(siB)
  [d_siB] -> Limiting_Acceleration/2(d_siB)
  siB_c/1 -> Saturation/1  "siB_c"
  Constant/1 -> Add2/1
  Add2/1 -> Saturation1/1
  Saturation/1 -> Add/1
  Integrator/1 -> Gain2/1, Limiting_Rate/2(d_siB)  "d_siB"
  Limiting_Rate/1(d_siB_l) -> Integrator1/1, [d_siB], d_siB/1  "d_siB_l"
  Limiting_Acceleration/1(dd_siB_l) -> dd_siB/1, Integrator/1  "dd_siB_l"
  Add/1 -> Gain/1
  Gain/1 -> Add1/1
  Gain2/1 -> Add1/2
  Add1/1 -> Limiting_Acceleration/3(dd_siB)  "dd_siB"
  Integrator1/1 -> Add/2, Gain1/1  "siB"
  tRRR/1 -> Sign/1  "tRRR"
  Sign/1 -> Gain3/1
  Gain3/1 -> Add2/3
  Gain1/1 -> Add2/2
  Integrator1/2 -> Integrator/2  "sat"
  Saturation1/1 -> [siB], siB/1  "siB"

== system lib_FDM/FDM/FDM_Sophisticated/fin_actuators/Rudder2 ==
  siB_c : Inport
  tRRR : Inport  Port=2
  Add : Sum  Inputs=+-
  Add1 : Sum  Inputs=+-
  Add2 : Sum  Inputs=+++
  Constant : Constant  Value=unc_off
  Gain : Gain  Gain=omega^2
  Gain1 : Gain  Gain=unc_scale
  Gain2 : Gain  Gain=2*dmp*omega  Multiplication=Matrix(K*u)
  Gain3 : Gain  Gain=unc_bl
  Integrator : Integrator  ExternalReset=either  InitialCondition=d_siB_0
  Integrator1 : Integrator  InitialCondition=siB_0  LimitOutput=on  UpperSaturationLimit=siB_max  LowerSaturationLimit=siB_min  ShowSaturationPort=on
  Limiting_Acceleration : MATLAB Function  TreatAsAtomicUnit=on
  Limiting_Rate : MATLAB Function  TreatAsAtomicUnit=on
  Saturation : Saturate  UpperLimit=siB_max  LowerLimit=siB_min
  Saturation1 : Saturate  UpperLimit=siB_max  LowerLimit=siB_min
  Sign : Signum
  siB : Outport  VectorParamsAs1DForOutWhenUnconnected=off
  d_siB : Outport  Port=2  VectorParamsAs1DForOutWhenUnconnected=off
  dd_siB : Outport  Port=3  VectorParamsAs1DForOutWhenUnconnected=off
  wires:
  [siB] -> Limiting_Rate/1(siB)
  [siB] -> Limiting_Acceleration/1(siB)
  [d_siB] -> Limiting_Acceleration/2(d_siB)
  siB_c/1 -> Saturation/1  "siB_c"
  Constant/1 -> Add2/1
  Add2/1 -> Saturation1/1
  Saturation/1 -> Add/1
  Integrator/1 -> Gain2/1, Limiting_Rate/2(d_siB)  "d_siB"
  Limiting_Rate/1(d_siB_l) -> Integrator1/1, [d_siB], d_siB/1  "d_siB_l"
  Limiting_Acceleration/1(dd_siB_l) -> dd_siB/1, Integrator/1  "dd_siB_l"
  Add/1 -> Gain/1
  Gain/1 -> Add1/1
  Gain2/1 -> Add1/2
  Add1/1 -> Limiting_Acceleration/3(dd_siB)  "dd_siB"
  Integrator1/1 -> Add/2, Gain1/1  "siB"
  tRRR/1 -> Sign/1  "tRRR"
  Sign/1 -> Gain3/1
  Gain3/1 -> Add2/3
  Gain1/1 -> Add2/2
  Integrator1/2 -> Integrator/2  "sat"
  Saturation1/1 -> [siB], siB/1  "siB"

== system lib_FDM/FDM/FDM_Sophisticated/fin_actuators/Rudder3 ==
  siB_c : Inport
  tRRR : Inport  Port=2
  Add : Sum  Inputs=+-
  Add1 : Sum  Inputs=+-
  Add2 : Sum  Inputs=+++
  Constant : Constant  Value=unc_off
  Gain : Gain  Gain=omega^2
  Gain1 : Gain  Gain=unc_scale
  Gain2 : Gain  Gain=2*dmp*omega  Multiplication=Matrix(K*u)
  Gain3 : Gain  Gain=unc_bl
  Integrator : Integrator  ExternalReset=either  InitialCondition=d_siB_0
  Integrator1 : Integrator  InitialCondition=siB_0  LimitOutput=on  UpperSaturationLimit=siB_max  LowerSaturationLimit=siB_min  ShowSaturationPort=on
  Limiting_Acceleration : MATLAB Function  TreatAsAtomicUnit=on
  Limiting_Rate : MATLAB Function  TreatAsAtomicUnit=on
  Saturation : Saturate  UpperLimit=siB_max  LowerLimit=siB_min
  Saturation1 : Saturate  UpperLimit=siB_max  LowerLimit=siB_min
  Sign : Signum
  siB : Outport  VectorParamsAs1DForOutWhenUnconnected=off
  d_siB : Outport  Port=2  VectorParamsAs1DForOutWhenUnconnected=off
  dd_siB : Outport  Port=3  VectorParamsAs1DForOutWhenUnconnected=off
  wires:
  [siB] -> Limiting_Rate/1(siB)
  [siB] -> Limiting_Acceleration/1(siB)
  [d_siB] -> Limiting_Acceleration/2(d_siB)
  siB_c/1 -> Saturation/1  "siB_c"
  Constant/1 -> Add2/1
  Add2/1 -> Saturation1/1
  Saturation/1 -> Add/1
  Integrator/1 -> Gain2/1, Limiting_Rate/2(d_siB)  "d_siB"
  Limiting_Rate/1(d_siB_l) -> Integrator1/1, [d_siB], d_siB/1  "d_siB_l"
  Limiting_Acceleration/1(dd_siB_l) -> dd_siB/1, Integrator/1  "dd_siB_l"
  Add/1 -> Gain/1
  Gain/1 -> Add1/1
  Gain2/1 -> Add1/2
  Add1/1 -> Limiting_Acceleration/3(dd_siB)  "dd_siB"
  Integrator1/1 -> Add/2, Gain1/1  "siB"
  tRRR/1 -> Sign/1  "tRRR"
  Sign/1 -> Gain3/1
  Gain3/1 -> Add2/3
  Gain1/1 -> Add2/2
  Integrator1/2 -> Integrator/2  "sat"
  Saturation1/1 -> [siB], siB/1  "siB"

== system lib_FDM/FDM/FDM_Sophisticated/fin_actuators/control_allocation ==
  siB : Inport
  d_siB : Inport  Port=2
  dd_siB : Inport  Port=3
  Constant8 : Constant  Value=HIL_Data.FDM.soph.bus1.Tr3r4
  Product : Product  Multiplication=Matrix(*)
  Product1 : Product  Multiplication=Matrix(*)
  Product2 : Product  Multiplication=Matrix(*)
  Tr3r4 : Outport  VectorParamsAs1DForOutWhenUnconnected=off
  finB : Outport  Port=2  VectorParamsAs1DForOutWhenUnconnected=off
  d_finB : Outport  Port=3  VectorParamsAs1DForOutWhenUnconnected=off
  dd_finB : Outport  Port=4  VectorParamsAs1DForOutWhenUnconnected=off
  wires:
  Product2/1 -> dd_finB/1  "dd_afinB"
  dd_siB/1 -> Product2/2
  Product1/1 -> d_finB/1  "d_afinB"
  d_siB/1 -> Product1/2
  siB/1 -> Product/2
  Constant8/1 -> Product/1, Product1/1, Product2/1, Tr3r4/1  "Tr3r4"
  Product/1 -> finB/1  "afinB"

== system lib_FDM/FDM/FDM_Sophisticated/gravity/launch_rail ==
  gBG_c : Inport
  hBE : Inport  Port=2
  Constant1 : Constant  Value=HIL_Data.FDM.soph.bus2.flag_I_gravity_switch
  Constant3 : Constant  Value=0
  Subtract : Sum  Inputs=++-
  Switch : Switch  Criteria=u2 > Threshold  Threshold=0.05
  Vector Concatenate : Concatenate  NumInputs=3
  initial_altitude : Subsystem
  gBG : Outport  VectorParamsAs1DForOutWhenUnconnected=off
  wires:
  initial_altitude/1(hBE_0) -> Subtract/3
  gBG_c/1 -> Switch/1
  Vector Concatenate/1 -> Switch/3
  Switch/1 -> gBG/1  "gBG"
  Constant3/1 -> Vector Concatenate/3, Vector Concatenate/2, Vector Concatenate/1
  Subtract/1 -> Switch/2
  hBE/1 -> Subtract/1
  Constant1/1 -> Subtract/2

== system lib_FDM/FDM/FDM_Sophisticated/motion_kinematics/calc_motion_kinematics ==
  lat : Inport
  lon : Inport  Port=2
  qIB : Inport  Port=3
  calc_transformation_matrix : Subsystem
  earth_rotation : Subsystem
  wIEE : Outport  VectorParamsAs1DForOutWhenUnconnected=off
  TIE : Outport  Port=2  VectorParamsAs1DForOutWhenUnconnected=off
  TEB : Outport  Port=3  VectorParamsAs1DForOutWhenUnconnected=off
  TGB : Outport  Port=4  VectorParamsAs1DForOutWhenUnconnected=off
  TEG : Outport  Port=5  VectorParamsAs1DForOutWhenUnconnected=off
  wEGG : Outport  Port=6  VectorParamsAs1DForOutWhenUnconnected=off
  TIB : Outport  Port=7  VectorParamsAs1DForOutWhenUnconnected=off
  wires:
  calc_transformation_matrix/3(TIB) -> TIB/1
  calc_transformation_matrix/2(TGB) -> TGB/1
  calc_transformation_matrix/1(TEB) -> TEB/1
  qIB/1 -> calc_transformation_matrix/3(qIB)
  earth_rotation/4(qEG) -> calc_transformation_matrix/2(qEG)
  earth_rotation/3(qIE) -> calc_transformation_matrix/1(qIE)
  lat/1 -> earth_rotation/1(lat)
  lon/1 -> earth_rotation/2(lon)
  earth_rotation/6(wEGG) -> wEGG/1
  earth_rotation/5(TEG) -> TEG/1
  earth_rotation/2(TIE) -> TIE/1
  earth_rotation/1(wIEE) -> wIEE/1

== system lib_FDM/FDM/FDM_Sophisticated/propulsion/prp_look_up ==
  env_glbl_bus : Inport
  Bus Selector1 : BusSelector  OutputSignals=T_sim_glbl,T_sim_lnch
  Constant : Constant  Value=0
  Constant1 : Constant  Value=0
  Saturation : Saturate  UpperLimit=HIL_Data.FDM.soph.bus1.t_prp1(end)  LowerLimit=0
      settings: AttributesFormatString=|
      | %<UpperLimit>
      | %<LowerLimit>
  Subtract : Sum  Inputs=+-
  Switch : Switch  Criteria=u2 > Threshold
  Switch1 : Switch  Criteria=u2 > Threshold
  Switch2 : Switch  Criteria=u2 > Threshold
  Vector Concatenate : Concatenate  NumInputs=3
  mass_flow_lookup : Lookup_n-D  NumberOfTableDimensions=1  BreakpointsForDimension1=HIL_Data.FDM.soph.bus1.d_mB.t_dmB  Table=HIL_Data.FDM.soph.bus1.d_mB.d_mB_lookup  ExtrapMethod=Clip  UseLastTableValue=on  InternalRulePriority=Speed  RndMeth=Simplest  InputSameDT=on
  thrust_lookup : Lookup_n-D  NumberOfTableDimensions=1  BreakpointsForDimension1=HIL_Data.FDM.soph.bus1.t_prp1  Table=HIL_Data.FDM.soph.bus1.F_prp  ExtrapMethod=Clip  UseLastTableValue=on  InternalRulePriority=Speed  RndMeth=Simplest  InputSameDT=on
  dmB : Outport  VectorParamsAs1DForOutWhenUnconnected=off
  FBPM : Outport  Port=2  VectorParamsAs1DForOutWhenUnconnected=off
  wires:
  Switch2/1 -> dmB/1  "dmB"
  mass_flow_lookup/1 -> Switch2/1
  Switch1/1 -> Vector Concatenate/1  "a_FBPM"
  Constant1/1 -> Vector Concatenate/2, Vector Concatenate/3
  Vector Concatenate/1 -> FBPM/1  "FBPM"
  Saturation/1 -> thrust_lookup/1, Switch2/3, Switch2/2, mass_flow_lookup/1
  Subtract/1 -> Switch/2, Switch/1
  Constant/1 -> Switch/3
  env_glbl_bus/1 -> Bus Selector1/1
  Bus Selector1/1 -> Subtract/1  "<T_sim_glbl>"
  thrust_lookup/1 -> Switch1/1
  Switch/1 -> Switch1/3, Switch1/2, Saturation/1
  Bus Selector1/2 -> Subtract/2  "<T_sim_lnch>"

== system lib_FDM/FDM/FDM_Sophisticated/propulsion/prp_uncertainty ==
  FBPM : Inport
  wab : Inport  Port=2
  3_rot_mat : Subsystem  mask(Rotation um 1, 2 oder 3 Achsen){rot_1=Rotation um z-Achse, rot_2=Rotation um y-Achse, rot_3=Rotation um x-Achse}
      mask prompts: rot_1 "1. Rotation"; rot_2 "2. Rotation"; rot_3 "3. Rotation"
      mask help:
      | Dieser Block liefert die Rotationsmatrix T12 für den Fall zurück, dass sich das Ziel-Koordinatensystem (1) durch Drehungen um 1, 2 oder 3 Achsen gegenüber dem Ausgangskoordinatensystem (2) beschreiben lässt (passive Drehung).
      |
      | Die Anzahl der Rotation sowie die Reihenfolge ist frei einstellbar.
      |
      | Die Rotationswinkel haben die Einheit [rad].
      mask TypeOptions rot_1: Rotation um x-Achse | Rotation um y-Achse | Rotation um z-Achse
      mask TypeOptions rot_2: Rotation um x-Achse | Rotation um y-Achse | Rotation um z-Achse
      mask TypeOptions rot_3: Rotation um x-Achse | Rotation um y-Achse | Rotation um z-Achse
  Bus Selector : BusSelector  OutputSignals=pBSB
  Product : Product  Multiplication=Matrix(*)
  Product1 : Product
  Subtract : Sum  Inputs=+-
  Thrust_rot_z : Constant  Value=HIL_Data.FDM.soph.bus1.unc_prp_z
  cross_product : Subsystem
      mask help: cross product r3 = r1 x r2
      mask Help:
      | Name:
      | 
      |     cross_product
      | 
      | Description:
      | 
      |     This block implements the cross product r3 = r1 x r2.
      | 
      | Inputs  [size] [data type] [unit]:
      | 
      |     vector 1  [3] [double] [-]
      |     vector 2  [3] [double] [-]
      | 
      | Outputs  [size] [data type] [unit]:
      | 
      |     resulting vector  [3] [double] [-]
      mask Display: disp(' r3 = r1 x r2')
  pNPB : Constant  Value=HIL_Data.FDM.soph.bus1.pNPB
  thrust_rot_x : Constant  Value=HIL_Data.FDM.soph.bus1.unc_prp_x
  thrust_rot_y : Constant  Value=HIL_Data.FDM.soph.bus1.unc_prp_y
  uncert_thrust : Constant  Value=HIL_Data.FDM.soph.bus1.unc_prp_scale
  FBPB : Outport  VectorParamsAs1DForOutWhenUnconnected=off
  MBPB : Outport  Port=2  VectorParamsAs1DForOutWhenUnconnected=off
  wires:
  Subtract/1 -> cross_product/1(r1)
  pNPB/1 -> Subtract/2
  Product1/1 -> Product/2
  uncert_thrust/1 -> Product1/2
  Bus Selector/1 -> Subtract/1  "<pBSB>"
  wab/1 -> Bus Selector/1
  cross_product/1(r1_x_r2) -> MBPB/1  "MBPB"
  thrust_rot_y/1 -> 3_rot_mat/2(wi2)
  3_rot_mat/1(T12) -> Product/1
  FBPM/1 -> Product1/1
  Product/1 -> FBPB/1, cross_product/2(r2)  "FBPB"
  thrust_rot_x/1 -> 3_rot_mat/3(wi3)
  Thrust_rot_z/1 -> 3_rot_mat/1(wi1)

== system lib_FDM/FDM/FDM_Sophisticated/rb_eom/calc_bus_flight_dyn_bus_entries ==
  mot_kin : Inport
  eom : Inport  Port=2
  Bus Selector : BusSelector  OutputSignals=pBII,vBII,qIB,wBIB,d_wBIB,d_vBII
  Bus Selector3 : BusSelector  OutputSignals=TIB,TIE
  Math Function : Math  Operator=transpose  SaturateOnIntegerOverflow=on
  Product : Product  Multiplication=Matrix(*)
  Product1 : Product  Multiplication=Matrix(*)
  Subsystem2 : Subsystem
  quaternion_to_euler_angles : Subsystem
      mask help: transforms quaternions to Euler angles (roll, pitch, yaw)
      mask Help:
      | Name:
      | 
      |     quaternion_to_euler_angles
      | 
      | Description:
      | 
      |     This block implements the transformation of a quaternion into the
      |     corresponding Euler angles (zyx-sequence, roll, pitch, yaw).
      | 
      | Inputs  [size] [data type] [unit]:
      | 
      |     quaternion  [4] [double] [-]
      | 
      | Outputs  [size] [data type] [unit]:
      | 
      |     roll angle phi  [1] [double] [rad]
      |     pitch angle theta  [1] [double] [rad]
      |     yaw angle psi  [1] [double] [rad]
      mask Display:
      | %disp (' q --> (Phi,Theta,Psi) [rad]')
      | disp('q \rightarrow eu(\Phi;\Theta;\Psi)','texmode','on')
  aBIB : Outport  VectorParamsAs1DForOutWhenUnconnected=off
  lon : Outport  Port=2  VectorParamsAs1DForOutWhenUnconnected=off
  lat : Outport  Port=3  VectorParamsAs1DForOutWhenUnconnected=off
  hBE : Outport  Port=4  VectorParamsAs1DForOutWhenUnconnected=off
  vBII : Outport  Port=5  VectorParamsAs1DForOutWhenUnconnected=off
  qIB : Outport  Port=6  VectorParamsAs1DForOutWhenUnconnected=off
  wBIB : Outport  Port=7  VectorParamsAs1DForOutWhenUnconnected=off
  d_wBIB : Outport  Port=8  VectorParamsAs1DForOutWhenUnconnected=off
  d_vBII : Outport  Port=9  VectorParamsAs1DForOutWhenUnconnected=off
  pBII : Outport  Port=10  VectorParamsAs1DForOutWhenUnconnected=off
  euIB : Outport  Port=11  VectorParamsAs1DForOutWhenUnconnected=off
  vBIB : Outport  Port=12  VectorParamsAs1DForOutWhenUnconnected=off
  wires:
  Product1/1 -> vBIB/1  "vBIB"
  quaternion_to_euler_angles/1(eulx) -> euIB/1  "euIB"
  Bus Selector/5 -> d_wBIB/1  "<d_wBIB>"
  Bus Selector/4 -> wBIB/1  "<wBIB>"
  Bus Selector/3 -> qIB/1, quaternion_to_euler_angles/1(q)  "<qIB>"
  Bus Selector/2 -> vBII/1, Product1/2  "<vBII>"
  Subsystem2/3(hBE) -> hBE/1  "hBE"
  Subsystem2/2(lat) -> lat/1
  Subsystem2/1(lon) -> lon/1
  Product/1 -> aBIB/1  "aBIB"
  Bus Selector/6 -> d_vBII/1, Product/2  "<d_vBII>"
  Bus Selector3/1 -> Math Function/1  "<TIB>"
  Math Function/1 -> Product/1, Product1/1  "TBI"
  eom/1 -> Bus Selector/1
  Bus Selector3/2 -> Subsystem2/1(TIE)  "<TIE>"
  mot_kin/1 -> Bus Selector3/1
  Bus Selector/1 -> Subsystem2/2(pBII), pBII/1  "<pBII>"

== system lib_FDM/FDM/FDM_Sophisticated/rb_eom/eom_6dof ==
  for_mom : Inport
  wab : Inport  Port=2
  Bus Selector1 : BusSelector  OutputSignals=mB,JBBB
  Bus Selector2 : BusSelector  OutputSignals=FBTB,MBTB
  Constant : Constant  Value=[HIL_Data.FDM.soph.bus2.pBII_0; HIL_Data.FDM.soph.bus2.vBII_0; HIL_Data.FDM.soph.bus2.qIB_0; HIL_Data.FDM.soph.bus2.wBIB_0]
  Constant9 : Constant  Value=[0 0 0; 0 0 0; 0 0 0]
  Rigid_Body_EOM_6_DOF : Subsystem  mask{flag_Kraft=FBTB}
      mask prompts: flag_Kraft "Input Kraftvektor"
      mask help:
      | 6DOF-Bewegungsgleichungen im ECI-System mit
      | zeitvariantem Massenträgheitsmoment.
      |
      | Modell Varianten:
      | - Koordinatensystem des Kraftvektor:
      |      FBTI : Inertial System I
      |      FBTB : Körperfestes System B
      mask init:
      | switch flag_Kraft
      |     case 1
      |         port_label_kraft = 'FBTI';
      |     case 2
      |         port_label_kraft = 'FBTB';
      | end
      mask TypeOptions flag_Kraft: FBTI | FBTB
      mask DialogControl Container4 Prompt: Modell Einstellungen
      mask Display:
      | port_label ('input',1,port_label_kraft )
      | port_label ('input',2,'MBTB' )
      | port_label ('input',3,'mB' )
      | port_label ('input',4,'x0' )
      | port_label ('input',5,'JBB' )
      | port_label ('input',6,'d_JBB' )
      | port_label ('output',1,'rb_eom' )
  eom : Outport  VectorParamsAs1DForOutWhenUnconnected=off
  wires:
  wab/1 -> Bus Selector1/1
  Bus Selector1/1 -> Rigid_Body_EOM_6_DOF/3(mB)  "<mB>"
  Constant/1 -> Rigid_Body_EOM_6_DOF/4(x0)
  for_mom/1 -> Bus Selector2/1
  Bus Selector1/2 -> Rigid_Body_EOM_6_DOF/5(JBB)  "<JBBB>"
  Constant9/1 -> Rigid_Body_EOM_6_DOF/6(d_JBB)
  Rigid_Body_EOM_6_DOF/1(rb_eom) -> eom/1
  Bus Selector2/1 -> Rigid_Body_EOM_6_DOF/1(FBTX)  "<FBTB>"
  Bus Selector2/2 -> Rigid_Body_EOM_6_DOF/2(MBTB)  "<MBTB>"

== system lib_FDM/FDM/FDM_Sophisticated/stream_flow/calc_stream_flow ==
  TIB : Inport
  wIEE : Inport  Port=2
  TIE : Inport  Port=3
  TGB : Inport  Port=4
  vBII : Inport  Port=5
  pBII : Inport  Port=6
  wBIB : Inport  Port=7
  rho : Inport  Port=8
  sos : Inport  Port=9
  hBE : Inport  Port=10
  vWEG : Inport  Port=11
  Bus Creator : BusCreator  Inputs=9
  Math Function : Math  Operator=transpose  SaturateOnIntegerOverflow=on
  Math Function1 : Math  Operator=transpose  SaturateOnIntegerOverflow=on
  Product : Product  Multiplication=Matrix(*)
  Product1 : Product  Multiplication=Matrix(*)
  Subsystem1 : Subsystem
  velocity_vector_transformation : Subsystem
  str_flow : Outport  VectorParamsAs1DForOutWhenUnconnected=off
  wires:
  Product1/1 -> Subsystem1/1(vWEB)  "vBEB_w"
  Math Function1/1 -> Product1/1  "TBG"
  vWEG/1 -> Product1/2
  TGB/1 -> Math Function1/1
  pBII/1 -> velocity_vector_transformation/4(pBII)
  TIB/1 -> Math Function/1
  rho/1 -> Subsystem1/4(rho)
  sos/1 -> Subsystem1/5(sos)
  hBE/1 -> Bus Creator/9
  wBIB/1 -> Subsystem1/3(wBIB)
  Bus Creator/1 -> str_flow/1  "str_flow_bus"
  wIEE/1 -> velocity_vector_transformation/1(wIEE)
  Subsystem1/1(al) -> Bus Creator/1  "alB"
  Subsystem1/7(th) -> Bus Creator/7  "inB"
  velocity_vector_transformation/1(vBEI) -> Product/2
  Subsystem1/3(qdynB) -> Bus Creator/3
  TIE/1 -> velocity_vector_transformation/2(TIE)
  Subsystem1/6(wBIB_star) -> Bus Creator/6
  Product/1 -> Subsystem1/2(vBEB)  "vBEB_k"
  Subsystem1/5(a_vB) -> Bus Creator/5
  vBII/1 -> velocity_vector_transformation/3(vBII)
  Subsystem1/8(fi) -> Bus Creator/8  "fiB"
  Subsystem1/2(be) -> Bus Creator/2  "beB"
  Math Function/1 -> Product/1  "TBI"
  Subsystem1/4(MaB) -> Bus Creator/4

== system lib_FDM/FDM/FDM_Sophisticated/tmp/Time ==
  Clock : Clock
  Constant6 : Constant  Value=HIL_Data.FDM.soph.bus2.T_sim_lnch
  T_sim_glbl : Outport  VectorParamsAs1DForOutWhenUnconnected=off
  T_sim_lnch : Outport  Port=2  VectorParamsAs1DForOutWhenUnconnected=off
  wires:
  Clock/1 -> T_sim_glbl/1  "T_sim_glbl"
  Constant6/1 -> T_sim_lnch/1  "T_sim_lnch"

== system lib_FDM/FDM/FDM_Sophisticated/tmp/weather ==
  atm_dynamic : Subsystem
  deviation_Tmp : Constant  Value=HIL_Data.FDM.soph.bus2.e_Tmp
  deviation_pa_QFH : Constant  Value=HIL_Data.FDM.soph.bus2.e_pa
  atm_dyn : Outport  VectorParamsAs1DForOutWhenUnconnected=off
  e_Tmp : Outport  Port=2  VectorParamsAs1DForOutWhenUnconnected=off
  e_pa : Outport  Port=3  VectorParamsAs1DForOutWhenUnconnected=off
  wires:
  deviation_pa_QFH/1 -> e_pa/1  "e_pa"
  atm_dynamic/1(vWEG) -> atm_dyn/1
  deviation_Tmp/1 -> e_Tmp/1  "e_Tmp"
